simulink model "RCL_simu"  (R2023b)
settings: Solver=FixedStepAuto  StartTime=0.0  StopTime=0.0005  FixedStep=0.000001  RelTol=1e-3
undefined symbols (not defined in the file or in its folder): C, L, R
settings Model: Creator=jerryling  LastModifiedBy=jerryling

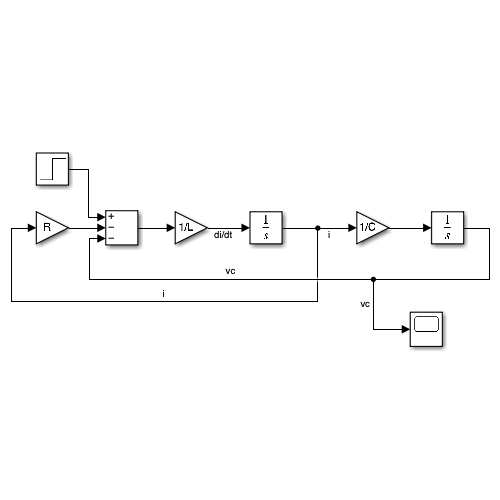
[thumbnail: Simulink's stored preview of the top-level diagram]
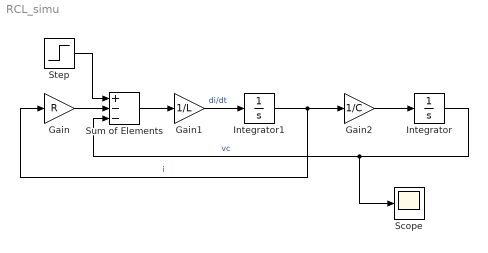
== system RCL_simu ==
  Gain : Gain  Gain=R
  Gain1 : Gain  Gain=1/L
  Gain2 : Gain  Gain=1/C
  Integrator : Integrator
  Integrator1 : Integrator
  Scope : Scope
  Step : Step  Time=0  After=5  SampleTime=0
  Sum of Elements : Sum  Inputs=+--
  wires:
  Step/1 -> Sum of Elements/1
  Gain/1 -> Sum of Elements/2
  Sum of Elements/1 -> Gain1/1
  Gain1/1 -> Integrator1/1  "di/dt"
  Integrator1/1 -> Gain/1, Gain2/1  "i"
  Gain2/1 -> Integrator/1
  Integrator/1 -> Scope/1, Sum of Elements/3  "vc"
